simulink model "Nominal_Receding_DO_CBF_ACC"  (R2018a)
settings: Solver=FixedStepAuto  StartTime=0.0  StopTime=Tsim  FixedStep=0.001  RelTol=1e-3
InitFcn:
  | tic;
  | disp('Simulation started...');
StopFcn:
  | elapsedTime_nominal_DO = toc; % Stop timer when simulation ends
  | fprintf('Simulation Time: %.6f seconds\n', elapsedTime_nominal_DO);
  | 
  | out_nominal_DO = out;
undefined symbols (not defined in the file): case_num, epsilon, f0, f1, f2, g, gamma, k, k_fric, m, magnitude, omega0, p_omega, psc, v0, vd
settings Model: Creator=Administrator  LastModifiedBy=Admin
settings DataIOCC: ReturnWorkspaceOutputs=on
settings SFSimCC: SimUseLocalCustomCode=on
settings RTWCC: RTWUseLocalCustomCode=on

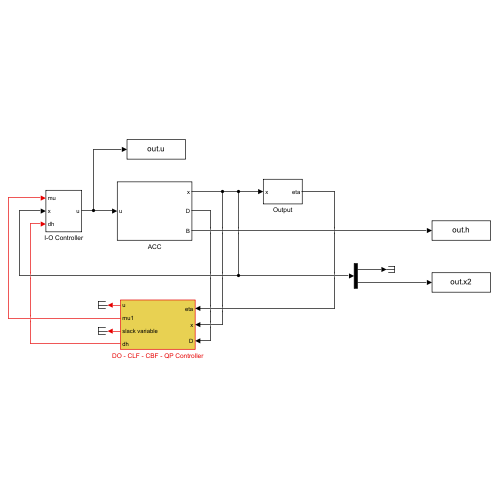
[thumbnail: Simulink's stored preview of the top-level diagram]
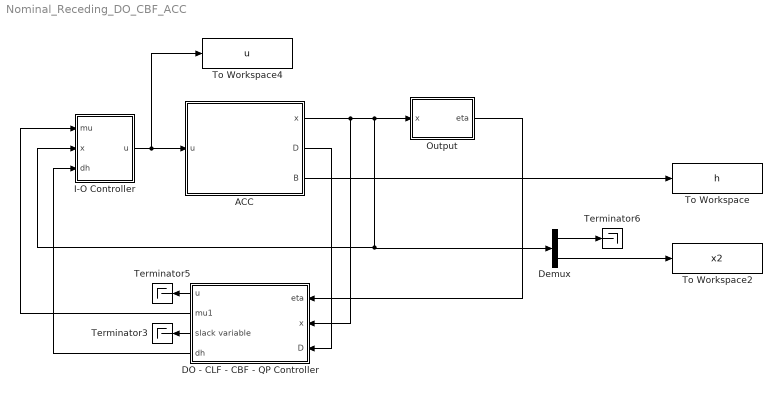
== system Nominal_Receding_DO_CBF_ACC ==
  ACC : Subsystem
  DO - CLF - CBF - QP Controller : Subsystem
  Demux : Demux  Outputs=2
  I-O Controller : Subsystem
  Output : Subsystem
  Terminator3 : Terminator
  Terminator5 : Terminator
  Terminator6 : Terminator
  To Workspace : ToWorkspace  VariableName=h  SampleTime=-1
  To Workspace2 : ToWorkspace  VariableName=x2  SampleTime=-1
  To Workspace4 : ToWorkspace  VariableName=u  SampleTime=-1
  wires:
  ACC/1(x) -> DO - CLF - CBF - QP Controller/2(x), I-O Controller/2(x), Demux/1, Output/1(x)
  I-O Controller/1(u) -> To Workspace4/1, ACC/1(u)
  DO - CLF - CBF - QP Controller/3(slack variable) -> Terminator3/1
  DO - CLF - CBF - QP Controller/1(u) -> Terminator5/1
  ACC/2(D) -> DO - CLF - CBF - QP Controller/3(D)
  Demux/1 -> Terminator6/1
  DO - CLF - CBF - QP Controller/2(mu1) -> I-O Controller/1(mu)
  Demux/2 -> To Workspace2/1
  Output/1(eta) -> DO - CLF - CBF - QP Controller/1(eta)
  ACC/3(B) -> To Workspace/1
  DO - CLF - CBF - QP Controller/4(dh) -> I-O Controller/3(dh)

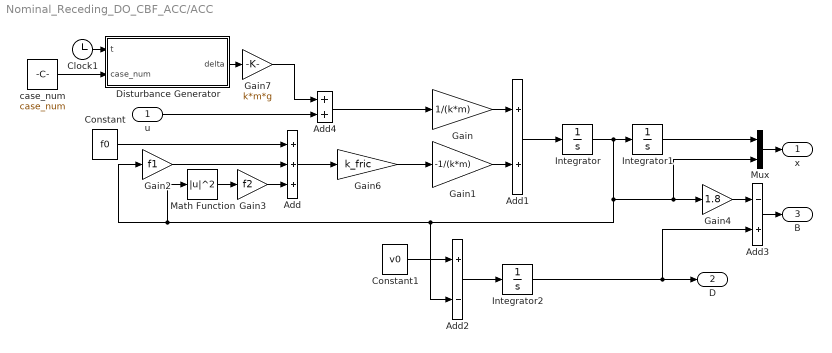
== system Nominal_Receding_DO_CBF_ACC/ACC ==
  u : Inport  PortDimensions=1
  Add : Sum  Inputs=+++
  Add1 : Sum
  Add2 : Sum  Inputs=+-
  Add3 : Sum  Inputs=-+
  Add4 : Sum
  Clock1 : Clock
  Constant : Constant  Value=f0
  Constant1 : Constant  Value=v0
  Disturbance Generator : MATLAB Function  TreatAsAtomicUnit=on
  Gain : Gain  Gain=1/(k*m)
  Gain1 : Gain  Gain=-1/(k*m)
  Gain2 : Gain  Gain=f1
  Gain3 : Gain  Gain=f2
  Gain4 : Gain  Gain=1.8
  Gain6 : Gain  Gain=k_fric
  Gain7 : Gain  Gain=k*m*g
  Integrator : Integrator  InitialCondition=20
  Integrator1 : Integrator
  Integrator2 : Integrator  InitialCondition=100
  Math Function : Math  Operator=magnitude^2  SaturateOnIntegerOverflow=on
  Mux : Mux  Inputs=2
  case_num : Constant  Value=case_num
  x : Outport  PortDimensions=2
  D : Outport  Port=2  PortDimensions=1
  B : Outport  Port=3  PortDimensions=1
  wires:
  Constant/1 -> Add/1
  Gain2/1 -> Add/2
  Gain3/1 -> Add/3
  Gain/1 -> Add1/1
  Gain1/1 -> Add1/2
  Add1/1 -> Integrator/1
  Integrator/1 -> Add2/2, Math Function/1, Gain2/1, Mux/2, Gain4/1, Integrator1/1
  Math Function/1 -> Gain3/1
  Constant1/1 -> Add2/1
  Add2/1 -> Integrator2/1
  Integrator2/1 -> Add3/2, D/1
  Gain4/1 -> Add3/1
  Add3/1 -> B/1
  Mux/1 -> x/1
  Integrator1/1 -> Mux/1
  Gain7/1 -> Add4/1
  Add4/1 -> Gain/1
  Add/1 -> Gain6/1
  Gain6/1 -> Gain1/1
  u/1 -> Add4/2
  Clock1/1 -> Disturbance Generator/1(t)
  case_num/1 -> Disturbance Generator/2(case_num)
  Disturbance Generator/1(delta) -> Gain7/1

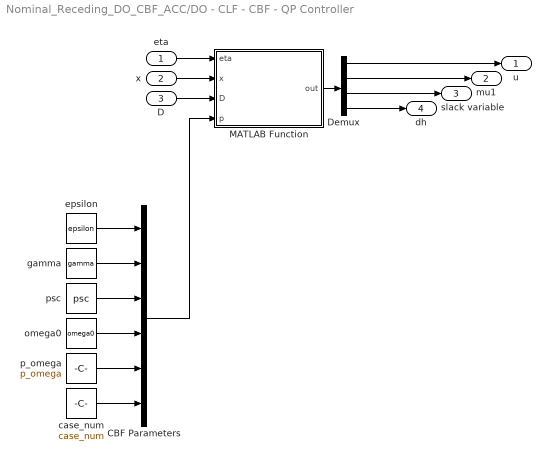
== system Nominal_Receding_DO_CBF_ACC/DO - CLF - CBF - QP Controller ==
  eta : Inport  PortDimensions=1
  x : Inport  Port=2  PortDimensions=2
  D : Inport  Port=3  PortDimensions=1
  CBF Parameters : Mux  Inputs=6
  Demux : Demux
  MATLAB Function : MATLAB Function  TreatAsAtomicUnit=on  SystemSampleTime=0.001
  case_num : Constant  Value=case_num
  epsilon : Constant  Value=epsilon
  gamma : Constant  Value=gamma
  omega0 : Constant  Value=omega0
  p_omega : Constant  Value=p_omega
  psc : Constant  Value=psc
  u : Outport  PortDimensions=1
  mu1 : Outport  Port=2  PortDimensions=1
  slack variable : Outport  Port=3  PortDimensions=1
  dh : Outport  Port=4  PortDimensions=1
  wires:
  Demux/3 -> slack variable/1
  eta/1 -> MATLAB Function/1(eta)
  D/1 -> MATLAB Function/3(D)
  Demux/2 -> mu1/1
  Demux/4 -> dh/1
  Demux/1 -> u/1
  x/1 -> MATLAB Function/2(x)
  MATLAB Function/1(out) -> Demux/1
  gamma/1 -> CBF Parameters/2
  omega0/1 -> CBF Parameters/4
  epsilon/1 -> CBF Parameters/1
  p_omega/1 -> CBF Parameters/5
  psc/1 -> CBF Parameters/3
  CBF Parameters/1 -> MATLAB Function/4(p)
  case_num/1 -> CBF Parameters/6

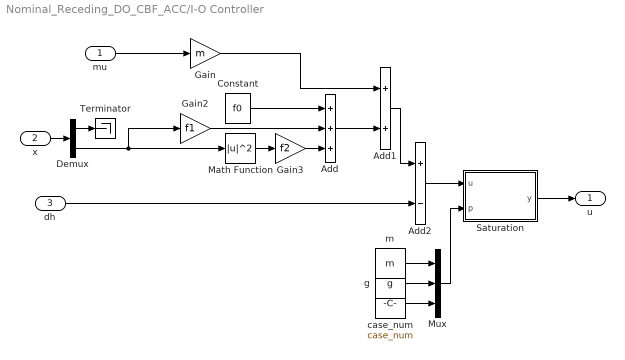
== system Nominal_Receding_DO_CBF_ACC/I-O Controller ==
  mu : Inport
  x : Inport  Port=2  PortDimensions=2
  dh : Inport  Port=3
  Add : Sum  Inputs=+++
  Add1 : Sum
  Add2 : Sum  Inputs=+-
  Constant : Constant  Value=f0
  Demux : Demux  Outputs=2
  Gain : Gain  Gain=m
  Gain2 : Gain  Gain=f1
  Gain3 : Gain  Gain=f2
  Math Function : Math  Operator=magnitude^2  SaturateOnIntegerOverflow=on
  Mux : Mux  Inputs=3
  Saturation : MATLAB Function  TreatAsAtomicUnit=on
  Terminator : Terminator
  case_num : Constant  Value=case_num
  g : Constant  Value=g
  m : Constant  Value=m
  u : Outport  PortDimensions=1
  wires:
  Gain3/1 -> Add/3
  Constant/1 -> Add/1
  Math Function/1 -> Gain3/1
  Gain2/1 -> Add/2
  Add/1 -> Add1/2
  mu/1 -> Gain/1
  Gain/1 -> Add1/1
  x/1 -> Demux/1
  Demux/2 -> Math Function/1, Gain2/1
  Demux/1 -> Terminator/1
  Add1/1 -> Add2/1
  Saturation/1(y) -> u/1
  dh/1 -> Add2/2
  Add2/1 -> Saturation/1(u)
  case_num/1 -> Mux/3
  Mux/1 -> Saturation/2(p)
  g/1 -> Mux/2
  m/1 -> Mux/1

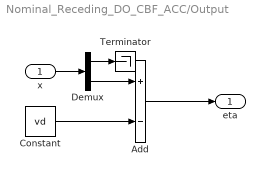
== system Nominal_Receding_DO_CBF_ACC/Output ==
  x : Inport  PortDimensions=2
  Add : Sum  Inputs=+-
  Constant : Constant  Value=vd
  Demux : Demux  Outputs=2
  Terminator : Terminator
  eta : Outport  PortDimensions=1
  wires:
  Constant/1 -> Add/2
  Add/1 -> eta/1
  Demux/2 -> Add/1
  x/1 -> Demux/1
  Demux/1 -> Terminator/1

== matlab function Nominal_Receding_DO_CBF_ACC/DO - CLF - CBF - QP Controller/MATLAB Function ==
  data: eta input; out output; x input; D input; p input
function out = DO_QP_Controller(eta, x, D, p)
coder.extrinsic('quadprog');
out = zeros(4,1);
persistent dh x0 x_hat0 u_qp

if isempty(dh),     dh     = 0; end
if isempty(x0),     x0     = [0; 20; 100]; end
if isempty(x_hat0), x_hat0 = [0; 0; 0]; end
if isempty(u_qp),   u_qp   = 0; end

case_num = p(6);
if case_num == 1 || case_num == 2
    mode = 1;
else 
    mode = 2;
end

dhExist = 1;
dhInputSubsetExist = 1;

x2 = x(2); 

%% Physical parameters
m = 1650;
g = 9.81; 
f0 = 0.1;
f1 = 5;
f2 = 0.25;
vd = 24;
v0 =  13.89;

ca = 0.3;
cd = 0.3;

%% Controller parameters
epsilon = p(1); 
gamma = p(2);
psc = p(3);
omega0 = p(4); 
p_omega = p(5);

Ts = 0.001;

%% Aerodynamic drag force
Fr = f0 + f1*x2 + f2*x2.^2;

%% Disturbance Observer
fx = [x0(2); -(1/m)*(f0 + f1*x0(2) + f2*x0(2)^2); v0 - x0(2)];
gx = [0; 1/m; 0];
Fx = x0 + Ts*fx;
Gx = Ts*gx;

fz = [x_hat0(2); -(1/m)*(f0 + f1*x_hat0(2) + f2*x_hat0(2)^2); v0 - x_hat0(2)];
Fz = x_hat0 + Ts*fz;

x_hat = Fz + Gx*(u_qp - dh);
dh = dhExist*((Gx'*Gx)\Gx')*([x; D] - x_hat - Fx + Fz);

x0 = [x; D]; x_hat0 = [x; D];

%% ============== QP 1 (No input saturation) ==============
if mode == 1
    %% CLF
    y = eta;
    V = y^2;
    LfV = 2*y*(-Fr/m); LgV = 2*y/m;
    A_clf = [LgV 0 -1]; b_clf = -LfV -epsilon*V;
    
    %% CBF
    B = D - 1.8*x2;
    LfB = v0 - x2 + 1.8*Fr/m;
    LgB = -1.8/m;
    A_cbf = [-LgB, 0, 0]; b_cbf = LfB + gamma*B;
    
    %% I-O L
    Lfy = -Fr/m; Lgy = 1/m;
    A_iol = [Lgy -1 0]; b_iol = - Lfy;
    
    %% QP
    A_ieq = [A_clf; A_cbf]; b_ieq = [b_clf; b_cbf];
    
    A_eq = A_iol; b_eq = b_iol;
    
    H_acc = [0, 0, 0; 0, 1, 0; 0, 0, psc];
    F_acc = [0; 0; 0];
    
    U = quadprog(H_acc, F_acc, A_ieq, b_ieq, A_eq, b_eq);
    
    out = [U([1 2 3]); dh];
    u_qp = U(1);
end
%% ============== QP 2 (Input saturation is considered but no optimal-decay variable is involved) ==============
if mode == 2
    %% CLF
    y = eta;
    V = y^2;
    LfV = 2*y*(-Fr/m); LgV = 2*y/m;
    A_clf = [LgV 0 -1]; b_clf = -LfV -epsilon*V;
    
    %% CBF
    B = D - 1.8*x2;
    LfB = v0 - x2 + 1.8*Fr/m;
    LgB = -1.8/m;
    A_cbf = [-LgB, 0, 0]; b_cbf = LfB + gamma*B;
    
    %% FC
    umax = ca*m*g + dhInputSubsetExist*dh; 
    umin = -cd*m*g + dhInputSubsetExist*dh;
    A_fc = [1, 0, 0; -1, 0, 0]; b_fc = [umax; -umin];
    
    %% I-O L
    Lfy = -Fr/m; Lgy = 1/m;
    A_iol = [Lgy -1 0]; b_iol = - Lfy;
    
    %% QP
%     A_ieq = [A_clf; A_cbf; A_cbf2; A_fc]; b_ieq = [b_clf; b_cbf; b_cbf2; b_fc];
    A_ieq = [A_clf; A_cbf; A_fc]; b_ieq = [b_clf; b_cbf; b_fc];
    % A_ieq = [A_clf; A_cbf]; b_ieq = [b_clf; b_cbf];
    
    A_eq = A_iol; b_eq = b_iol;
    
    H_acc = [0, 0, 0; 0, 1, 0; 0, 0, psc];
    F_acc = [0; 0; 0];
    
    U = quadprog(H_acc, F_acc, A_ieq, b_ieq, A_eq, b_eq);
    
    out = [U([1 2 3]); dh];
    u_qp = U(1);
end


end

== matlab function Nominal_Receding_DO_CBF_ACC/I-O Controller/Saturation ==
  data: u input; y output; p input
function y = fcn(u, p)

m = p(1);
g = p(2);
case_num = p(3);

if case_num == 1 || case_num == 2
    y = u;
else
    if u >= 0.3*m*g
        y = 0.3*m*g;
    elseif u <= -0.3*m*g
        y = -0.3*m*g;
    else
        y = u;
    end
end

end

== matlab function Nominal_Receding_DO_CBF_ACC/ACC/Disturbance Generator ==
  data: t input; delta output; case_num input
function delta = fcn(t, case_num)

if case_num == 1
    delta = 0.16*cos(2*pi*t/20) + 0.14*sin(2*pi*t/10 + pi/3);
elseif case_num == 2
    delta = 0.16*cos(2*pi*t/20) + 0.14*sin(2*pi*t/10 + pi/3);
else
    % delta = 0.18*cos(2*pi*t/20) + 0.14*sin(2*pi*t/10 - pi/8);
    delta = -(0.12*cos(2*pi*t/20) + 0.08*sin(2*pi*t/10 + pi/3));
end
